simulink model "H175_PANKL_V1a_controlled_R2022b"  (R2022b)
settings: Solver=ode15s  StartTime=0.0  StopTime=22136  RelTol=1e-3  AbsTol=1e-3
PreLoadFcn:
  | omega_TLU = [1000, 1500, 2000, 2500, 3000, 3500];
  | beta_TLU = linspace(0,1,7);
  | 
  | mdot_TLU = [0.1377    0.1304    0.1187    0.1029    0.0854    0.0658    0.0437
  |     0.2310    0.2183    0.1978    0.1688    0.1400    0.1118    0.0750
  |     0.3298    0.3208    0.2987    0.2677    0.2256    0.1774    0.1194
  |     0.4520    0.4260    0.3825    0.3308    0.2745    0.2227    0.1655
  |     0.5542    0.5353    0.4781    0.4230    0.3477    0.2897    0.2211
  |     0.6197    0.5805    0.5198    0.4516    0.3971    0.3555    0.2825];
  | 
  | eta_TLU = [0.7905    0.8025    0.7998    0.7972    0.7932    0.7882    0.7827
  |     0.7993    0.8239    0.8350    0.8379    0.8197    0.8000    0.7809
  |     0.8011    0.8374    0.8632    0.8827    0.8749    0.8394    0.7948
  |     0.8072    0.8520    0.8814    0.9000    0.8676    0.8356    0.7971
  |     0.8076    0.8271    0.8608    0.8766    0.8529    0.8329    0.7992
  |     0.7949    0.8131    0.8296    0.8243    0.8170    0.8085    0.7972];
  | 
  | pr_TLU = [1.0912    1.1795    1.2293    1.2662    1.2928    1.3108    1.3151
  |     1.1484    1.3081    1.3958    1.4707    1.5136    1.5380    1.5456
  |     1.2830    1.4539    1.5943    1.7042    1.7973    1.8582    1.8799
  |     1.5180    1.8034    1.9693    2.0899    2.1662    2.2027    2.2182
  |     1.8359    2.0956    2.3359    2.4668    2.5687    2.6106    2.6224
  |     2.3061    2.6623    2.8585    2.9837    3.0443    3.0714    3.0869];
values from neighbouring files (symbols this model uses):
  P64_omega_TLU = [44762 68636 92509 110414 125335 137271 146224]    [All_Properties.mat]    (also in PANKL_CMP.mat = [44762 68636 92509 110414 125335 137271 146224 155176.0695 1)
libraries: fl_lib x101, nesl_utility x76, SimscapeFluids_lib x5, slpidlib x3
(part 4 of 4)

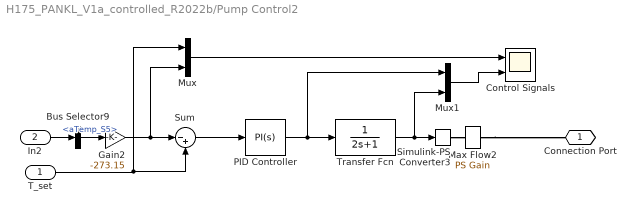
== system H175_PANKL_V1a_controlled_R2022b/Pump Control2 ==
  T_set : Inport
  In2 : Inport  Port=2
  Bus Selector9 : BusSelector  OutputSignals=aTemp_S5
  Control Signals : Scope  NumInputPorts=2
  Gain2 : Gain  Gain=-273.15
  Max Flow2 : fl_lib/Physical Signals/Functions/PS Gain  gain=2 kg/s
  Mux : Mux  Inputs=2
  Mux1 : Mux  Inputs=2
  PID Controller : slpidlib/PID Controller  Controller=PI  Form=Ideal  TimeDomain=Continuous-time  UseExternalTs=off  SampleTime=-1  IntegratorMethod=Forward Euler  FilterMethod=Forward Euler  ControllerParametersSource=internal  P=0.1  I=0.01  UseKiTs=off  D=0  N=100  UseFilter=on  TunerSelectOption=Transfer Function Based (PID Tuner App)  ZeroCross=off  InitialConditionSource=internal  InitialConditionForIntegrator=0  InitialConditionForFilter=0  DifferentiatorICPrevScaledInput=0  ExternalReset=none  TrackingMode=off  Kt=1  LimitOutput=on  SatLimitsSource=internal  UpperSaturationLimit=1  LowerSaturationLimit=0  LinearizeAsGain=on  AntiWindupMode=clamping  Kb=1  LimitIntegrator=off  UpperIntegratorSaturationLimit=inf  LowerIntegratorSaturationLimit=-inf  POutMin=[]  POutMax=[]  IOutMin=[]  IOutMax=[]  DOutMin=[]  DOutMax=[]  NOutMin=[]  NOutMax=[]  SumOutMin=[]  SumOutMax=[]  SaturationOutMin=[]  SaturationOutMax=[]  PParamMin=[]  PParamMax=[]  IParamMin=[]  IParamMax=[]  DParamMin=[]  DParamMax=[]  NParamMin=[]  NParamMax=[]  KbParamMin=[]  KbParamMax=[]  KtParamMin=[]  KtParamMax=[]  KbOutMin=[]  KbOutMax=[]  KtOutMin=[]  KtOutMax=[]  IntegratorOutMin=[]  IntegratorOutMax=[]  FilterOutMin=[]  FilterOutMax=[]  SumI1OutMin=[]  SumI1OutMax=[]  SumI2OutMin=[]  SumI2OutMax=[]  SumI3OutMin=[]  SumI3OutMax=[]  SumI4OutMin=[]  SumI4OutMax=[]  SumDOutMin=[]  SumDOutMax=[]  DifferentiatorOutMin=[]  DifferentiatorOutMax=[]  FilterDiffOutCoefMin=[]  FilterDiffOutCoefMax=[]  ReciprocalOutMin=[]  ReciprocalOutMax=[]  SumDenOutMin=[]  SumDenOutMax=[]  SumNumOutMin=[]  SumNumOutMax=[]  DivideOutMin=[]  DivideOutMax=[]  UdiffTsProdOutMin=[]  UdiffTsProdOutMax=[]  NTsProdOutMin=[]  NTsProdOutMax=[]  UintegralTsProdOutMin=[]  UintegralTsProdOutMax=[]  UngainTsProdOutMin=[]  UngainTsProdOutMax=[]  IntegratorContinuousStateAttributes=''  IntegratorStateMustResolveToSignalObject=off  IntegratorRTWStateStorageClass=Auto  FilterContinuousStateAttributes=''  FilterStateMustResolveToSignalObject=off  FilterRTWStateStorageClass=Auto  ParallelPVariant=Passthrough  IdealPVariant=InternalParameters  IVariant=InternalParameters  DVariant=Disabled  IntegratorVariant=Continuous  SatVariant=Enabled  AWVariant=ContClampingIdeal  PCopyVariant=InternalParamsIdeal  TRVariant=Disabled  FdbkBlocksVariant=Forward  IdealPFdbkVariant=Disabled  SatFdbkVariant=Disabled  DerivativeFilterVariant=Disabled  NVariant=Disabled  NCopyVariant=Disabled_SignalSpec  FilterICVariant=Disabled  IntegratorICVariant=InternalICs  ExternalResetVariant=Disabled  TRSumVariant=Passthrough  SumFdbkVariant=Disabled  SumVariant=Sum_PI  TsampFilterVariant=InternalTs  TsampNgainVariant=Passthrough  TsampIntegralVariant=Disabled_SignalSpec  ExternalSaturationOutDataTypeStr=Inherit: Same as second input
  Simulink-PS Converter3 : nesl_utility/Simulink-PS Converter  PhysicalDomain=network_engine_domain  SubClassName=ps_input  LeftPortType=input  RightPortType=output  PseudoPeriodic=off  Frequencies=[]  NoiseDistribution=none  NoiseParameters=[]  Unit=1  AffineConversion=off  FilteringAndDerivatives=provide  SimscapeFilterOrder=1  InputFilterTimeConstant=0.001  UdotUserProvided=0
  Sum : Sum  Inputs=|-+
  Transfer Fcn : TransferFcn  Denominator=[2 1]
  Connection Port : PMIOPort  Side=Right
  wires:
  Transfer Fcn/1 -> Simulink-PS Converter3/1, Mux1/2
  T_set/1 -> Mux/1, Sum/2
  Gain2/1 -> Sum/1, Mux/2
  Sum/1 -> PID Controller/1
  PID Controller/1 -> Mux1/1, Transfer Fcn/1
  Mux/1 -> Control Signals/1
  Mux1/1 -> Control Signals/2
  Bus Selector9/1 -> Gain2/1  "<aTemp_S5>"
  In2/1 -> Bus Selector9/1
  connections:
  Max Flow2/RConn1 -- Connection Port/RConn1
  Simulink-PS Converter3/RConn1 -- Max Flow2/LConn1

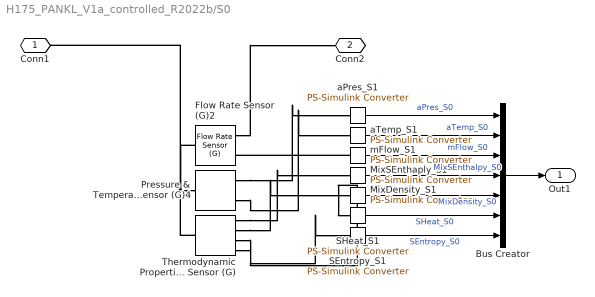
== system H175_PANKL_V1a_controlled_R2022b/S0 ==
  Bus Creator : BusCreator  Inputs=7
  Flow Rate Sensor (G)2 : fl_lib/Gas/Sensors/Flow Rate Sensor (G)  mass_flow_measure=true  volumetric_flow_measure=false  volumetric_flow_conditions=foundation.enum.volumetric_flow_conditions.actual  p_std=0.101325 MPa  T_std=20 degC  energy_flow_measure=false
      settings: InternalSimscapePortConfiguration="{\"Bottom\":[],\"Left\":[{\"id\":\"A\",\"label\":\"A\",\"type\":\"foundation.gas.gas\"}],\"Right\":[{\"id\":\"B\",\"label\":\"B\",\"type\":\"foundation.gas.gas\"},{\"id\":\"M\",\"label\":\"M\",\"type\":\"output\"}],\"Top\":[]}"
  MixDensity_S1 : nesl_utility/PS-Simulink Converter  PhysicalDomain=network_engine_domain  SubClassName=ps_output  LeftPortType=input  RightPortType=output  PseudoPeriodic=off  Frequencies=[]  VectorFormat=inherit  Unit=inherit  AffineConversion=off
  MixSEnthaply_S1 : nesl_utility/PS-Simulink Converter  PhysicalDomain=network_engine_domain  SubClassName=ps_output  LeftPortType=input  RightPortType=output  PseudoPeriodic=off  Frequencies=[]  VectorFormat=inherit  Unit=inherit  AffineConversion=off
  Pressure & Temperature Sensor (G)4 : fl_lib/Gas/Sensors/Pressure & Temperature Sensor (G)  reference=foundation.enum.MeasurementReference.absolute  pressure=true  pressure_spec=foundation.enum.PressureMeasementSpec.Absolute  temperature=true
      settings: InternalSimscapePortConfiguration="{\"Bottom\":[{\"id\":\"T\",\"label\":\"T\",\"type\":\"output\"}],\"Left\":[{\"id\":\"A\",\"label\":\"A\",\"type\":\"foundation.gas.gas\"}],\"Right\":[{\"id\":\"Pa\",\"label\":\"Pa\",\"type\":\"output\"}],\"Top\":[]}"
  SEntropy_S1 : nesl_utility/PS-Simulink Converter  PhysicalDomain=network_engine_domain  SubClassName=ps_output  LeftPortType=input  RightPortType=output  PseudoPeriodic=off  Frequencies=[]  VectorFormat=inherit  Unit=inherit  AffineConversion=off
  SHeat_S1 : nesl_utility/PS-Simulink Converter  PhysicalDomain=network_engine_domain  SubClassName=ps_output  LeftPortType=input  RightPortType=output  PseudoPeriodic=off  Frequencies=[]  VectorFormat=inherit  Unit=inherit  AffineConversion=off
  Thermodynamic Properties Sensor (G) : fl_lib/Gas/Sensors/Thermodynamic Properties Sensor (G)  enthalpy=true  density=true  specific_heat=true  entropy=true  s_std=3.8635 kJ/(K*kg)  p_std=0.101325 MPa  T_std=293.15 K
      settings: InternalSimscapePortConfiguration="{\"Bottom\":[{\"id\":\"CP\",\"label\":\"cp\",\"type\":\"output\"},{\"id\":\"S\",\"label\":\"s\",\"type\":\"output\"}],\"Left\":[{\"id\":\"A\",\"label\":\"A\",\"type\":\"foundation.gas.gas\"}],\"Right\":[{\"id\":\"H\",\"label\":\"h\",\"type\":\"output\"},{\"id\":\"RHO\",\"label\":\"ρ\",\"type\":\"output\"}],\"Top\":[]}"
  aPres_S1 : nesl_utility/PS-Simulink Converter  PhysicalDomain=network_engine_domain  SubClassName=ps_output  LeftPortType=input  RightPortType=output  PseudoPeriodic=off  Frequencies=[]  VectorFormat=inherit  Unit=inherit  AffineConversion=off
  aTemp_S1 : nesl_utility/PS-Simulink Converter  PhysicalDomain=network_engine_domain  SubClassName=ps_output  LeftPortType=input  RightPortType=output  PseudoPeriodic=off  Frequencies=[]  VectorFormat=inherit  Unit=degC  AffineConversion=off
  mFlow_S1 : nesl_utility/PS-Simulink Converter  PhysicalDomain=network_engine_domain  SubClassName=ps_output  LeftPortType=input  RightPortType=output  PseudoPeriodic=off  Frequencies=[]  VectorFormat=inherit  Unit=inherit  AffineConversion=off
  Conn1 : PMIOPort  Side=Left
  Conn2 : PMIOPort  Port=2  Side=Right
  Out1 : Outport
  wires:
  MixDensity_S1/1 -> Bus Creator/5  "MixDensity_S0"
  MixSEnthaply_S1/1 -> Bus Creator/4  "MixSEnthalpy_S0"
  mFlow_S1/1 -> Bus Creator/3  "mFlow_S0"
  Bus Creator/1 -> Out1/1
  aPres_S1/1 -> Bus Creator/1  "aPres_S0"
  SHeat_S1/1 -> Bus Creator/6  "SHeat_S0"
  SEntropy_S1/1 -> Bus Creator/7  "SEntropy_S0"
  aTemp_S1/1 -> Bus Creator/2  "aTemp_S0"
  connections:
  Flow Rate Sensor (G)2/RConn1 -- Conn2/RConn1
  Pressure & Temperature Sensor (G)4/RConn2 -- aTemp_S1/LConn1
  mFlow_S1/LConn1 -- Flow Rate Sensor (G)2/RConn2
  Thermodynamic Properties Sensor (G)/RConn1 -- MixSEnthaply_S1/LConn1
  Thermodynamic Properties Sensor (G)/RConn4 -- SEntropy_S1/LConn1
  Thermodynamic Properties Sensor (G)/RConn2 -- MixDensity_S1/LConn1
  Pressure & Temperature Sensor (G)4/RConn1 -- aPres_S1/LConn1
  Pressure & Temperature Sensor (G)4/LConn1 -- Thermodynamic Properties Sensor (G)/LConn1 -- Conn1/RConn1 -- Flow Rate Sensor (G)2/LConn1
  Thermodynamic Properties Sensor (G)/RConn3 -- SHeat_S1/LConn1

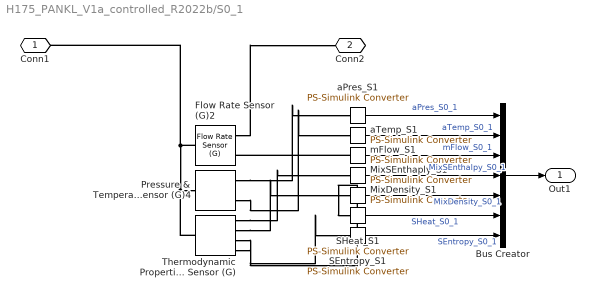
== system H175_PANKL_V1a_controlled_R2022b/S0_1 ==
  Bus Creator : BusCreator  Inputs=7
  Flow Rate Sensor (G)2 : fl_lib/Gas/Sensors/Flow Rate Sensor (G)  mass_flow_measure=true  volumetric_flow_measure=false  volumetric_flow_conditions=foundation.enum.volumetric_flow_conditions.actual  p_std=0.101325 MPa  T_std=20 degC  energy_flow_measure=false
      settings: InternalSimscapePortConfiguration="{\"Bottom\":[],\"Left\":[{\"id\":\"A\",\"label\":\"A\",\"type\":\"foundation.gas.gas\"}],\"Right\":[{\"id\":\"B\",\"label\":\"B\",\"type\":\"foundation.gas.gas\"},{\"id\":\"M\",\"label\":\"M\",\"type\":\"output\"}],\"Top\":[]}"
  MixDensity_S1 : nesl_utility/PS-Simulink Converter  PhysicalDomain=network_engine_domain  SubClassName=ps_output  LeftPortType=input  RightPortType=output  PseudoPeriodic=off  Frequencies=[]  VectorFormat=inherit  Unit=inherit  AffineConversion=off
  MixSEnthaply_S1 : nesl_utility/PS-Simulink Converter  PhysicalDomain=network_engine_domain  SubClassName=ps_output  LeftPortType=input  RightPortType=output  PseudoPeriodic=off  Frequencies=[]  VectorFormat=inherit  Unit=inherit  AffineConversion=off
  Pressure & Temperature Sensor (G)4 : fl_lib/Gas/Sensors/Pressure & Temperature Sensor (G)  reference=foundation.enum.MeasurementReference.absolute  pressure=true  pressure_spec=foundation.enum.PressureMeasementSpec.Absolute  temperature=true
      settings: InternalSimscapePortConfiguration="{\"Bottom\":[{\"id\":\"T\",\"label\":\"T\",\"type\":\"output\"}],\"Left\":[{\"id\":\"A\",\"label\":\"A\",\"type\":\"foundation.gas.gas\"}],\"Right\":[{\"id\":\"Pa\",\"label\":\"Pa\",\"type\":\"output\"}],\"Top\":[]}"
  SEntropy_S1 : nesl_utility/PS-Simulink Converter  PhysicalDomain=network_engine_domain  SubClassName=ps_output  LeftPortType=input  RightPortType=output  PseudoPeriodic=off  Frequencies=[]  VectorFormat=inherit  Unit=inherit  AffineConversion=off
  SHeat_S1 : nesl_utility/PS-Simulink Converter  PhysicalDomain=network_engine_domain  SubClassName=ps_output  LeftPortType=input  RightPortType=output  PseudoPeriodic=off  Frequencies=[]  VectorFormat=inherit  Unit=inherit  AffineConversion=off
  Thermodynamic Properties Sensor (G) : fl_lib/Gas/Sensors/Thermodynamic Properties Sensor (G)  enthalpy=true  density=true  specific_heat=true  entropy=true  s_std=3.8635 kJ/(K*kg)  p_std=0.101325 MPa  T_std=293.15 K
      settings: InternalSimscapePortConfiguration="{\"Bottom\":[{\"id\":\"CP\",\"label\":\"cp\",\"type\":\"output\"},{\"id\":\"S\",\"label\":\"s\",\"type\":\"output\"}],\"Left\":[{\"id\":\"A\",\"label\":\"A\",\"type\":\"foundation.gas.gas\"}],\"Right\":[{\"id\":\"H\",\"label\":\"h\",\"type\":\"output\"},{\"id\":\"RHO\",\"label\":\"ρ\",\"type\":\"output\"}],\"Top\":[]}"
  aPres_S1 : nesl_utility/PS-Simulink Converter  PhysicalDomain=network_engine_domain  SubClassName=ps_output  LeftPortType=input  RightPortType=output  PseudoPeriodic=off  Frequencies=[]  VectorFormat=inherit  Unit=inherit  AffineConversion=off
  aTemp_S1 : nesl_utility/PS-Simulink Converter  PhysicalDomain=network_engine_domain  SubClassName=ps_output  LeftPortType=input  RightPortType=output  PseudoPeriodic=off  Frequencies=[]  VectorFormat=inherit  Unit=degC  AffineConversion=off
  mFlow_S1 : nesl_utility/PS-Simulink Converter  PhysicalDomain=network_engine_domain  SubClassName=ps_output  LeftPortType=input  RightPortType=output  PseudoPeriodic=off  Frequencies=[]  VectorFormat=inherit  Unit=inherit  AffineConversion=off
  Conn1 : PMIOPort  Side=Left
  Conn2 : PMIOPort  Port=2  Side=Right
  Out1 : Outport
  wires:
  MixDensity_S1/1 -> Bus Creator/5  "MixDensity_S0_1"
  MixSEnthaply_S1/1 -> Bus Creator/4  "MixSEnthalpy_S0_1"
  mFlow_S1/1 -> Bus Creator/3  "mFlow_S0_1"
  Bus Creator/1 -> Out1/1
  aPres_S1/1 -> Bus Creator/1  "aPres_S0_1"
  SHeat_S1/1 -> Bus Creator/6  "SHeat_S0_1"
  SEntropy_S1/1 -> Bus Creator/7  "SEntropy_S0_1"
  aTemp_S1/1 -> Bus Creator/2  "aTemp_S0_1"
  connections:
  Flow Rate Sensor (G)2/RConn1 -- Conn2/RConn1
  Pressure & Temperature Sensor (G)4/RConn2 -- aTemp_S1/LConn1
  mFlow_S1/LConn1 -- Flow Rate Sensor (G)2/RConn2
  Thermodynamic Properties Sensor (G)/RConn1 -- MixSEnthaply_S1/LConn1
  Thermodynamic Properties Sensor (G)/RConn4 -- SEntropy_S1/LConn1
  Thermodynamic Properties Sensor (G)/RConn2 -- MixDensity_S1/LConn1
  Pressure & Temperature Sensor (G)4/RConn1 -- aPres_S1/LConn1
  Conn1/RConn1 -- Flow Rate Sensor (G)2/LConn1 -- Pressure & Temperature Sensor (G)4/LConn1 -- Thermodynamic Properties Sensor (G)/LConn1
  Thermodynamic Properties Sensor (G)/RConn3 -- SHeat_S1/LConn1

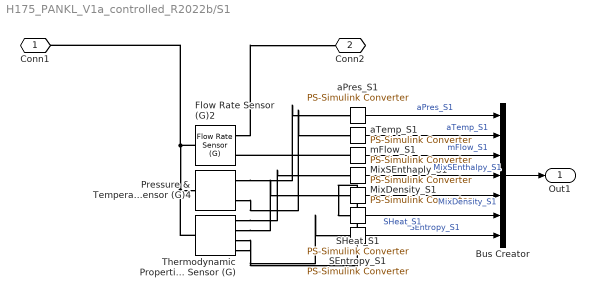
== system H175_PANKL_V1a_controlled_R2022b/S1 ==
  Bus Creator : BusCreator  Inputs=7
  Flow Rate Sensor (G)2 : fl_lib/Gas/Sensors/Flow Rate Sensor (G)  mass_flow_measure=true  volumetric_flow_measure=false  volumetric_flow_conditions=foundation.enum.volumetric_flow_conditions.actual  p_std=0.101325 MPa  T_std=20 degC  energy_flow_measure=false
      settings: InternalSimscapePortConfiguration="{\"Bottom\":[],\"Left\":[{\"id\":\"A\",\"label\":\"A\",\"type\":\"foundation.gas.gas\"}],\"Right\":[{\"id\":\"B\",\"label\":\"B\",\"type\":\"foundation.gas.gas\"},{\"id\":\"M\",\"label\":\"M\",\"type\":\"output\"}],\"Top\":[]}"
  MixDensity_S1 : nesl_utility/PS-Simulink Converter  PhysicalDomain=network_engine_domain  SubClassName=ps_output  LeftPortType=input  RightPortType=output  PseudoPeriodic=off  Frequencies=[]  VectorFormat=inherit  Unit=inherit  AffineConversion=off
  MixSEnthaply_S1 : nesl_utility/PS-Simulink Converter  PhysicalDomain=network_engine_domain  SubClassName=ps_output  LeftPortType=input  RightPortType=output  PseudoPeriodic=off  Frequencies=[]  VectorFormat=inherit  Unit=inherit  AffineConversion=off
  Pressure & Temperature Sensor (G)4 : fl_lib/Gas/Sensors/Pressure & Temperature Sensor (G)  reference=foundation.enum.MeasurementReference.absolute  pressure=true  pressure_spec=foundation.enum.PressureMeasementSpec.Absolute  temperature=true
      settings: InternalSimscapePortConfiguration="{\"Bottom\":[{\"id\":\"T\",\"label\":\"T\",\"type\":\"output\"}],\"Left\":[{\"id\":\"A\",\"label\":\"A\",\"type\":\"foundation.gas.gas\"}],\"Right\":[{\"id\":\"Pa\",\"label\":\"Pa\",\"type\":\"output\"}],\"Top\":[]}"
  SEntropy_S1 : nesl_utility/PS-Simulink Converter  PhysicalDomain=network_engine_domain  SubClassName=ps_output  LeftPortType=input  RightPortType=output  PseudoPeriodic=off  Frequencies=[]  VectorFormat=inherit  Unit=inherit  AffineConversion=off
  SHeat_S1 : nesl_utility/PS-Simulink Converter  PhysicalDomain=network_engine_domain  SubClassName=ps_output  LeftPortType=input  RightPortType=output  PseudoPeriodic=off  Frequencies=[]  VectorFormat=inherit  Unit=inherit  AffineConversion=off
  Thermodynamic Properties Sensor (G) : fl_lib/Gas/Sensors/Thermodynamic Properties Sensor (G)  enthalpy=true  density=true  specific_heat=true  entropy=true  s_std=3.8635 kJ/(K*kg)  p_std=0.101325 MPa  T_std=293.15 K
      settings: InternalSimscapePortConfiguration="{\"Bottom\":[{\"id\":\"CP\",\"label\":\"cp\",\"type\":\"output\"},{\"id\":\"S\",\"label\":\"s\",\"type\":\"output\"}],\"Left\":[{\"id\":\"A\",\"label\":\"A\",\"type\":\"foundation.gas.gas\"}],\"Right\":[{\"id\":\"H\",\"label\":\"h\",\"type\":\"output\"},{\"id\":\"RHO\",\"label\":\"ρ\",\"type\":\"output\"}],\"Top\":[]}"
  aPres_S1 : nesl_utility/PS-Simulink Converter  PhysicalDomain=network_engine_domain  SubClassName=ps_output  LeftPortType=input  RightPortType=output  PseudoPeriodic=off  Frequencies=[]  VectorFormat=inherit  Unit=inherit  AffineConversion=off
  aTemp_S1 : nesl_utility/PS-Simulink Converter  PhysicalDomain=network_engine_domain  SubClassName=ps_output  LeftPortType=input  RightPortType=output  PseudoPeriodic=off  Frequencies=[]  VectorFormat=inherit  Unit=degC  AffineConversion=off
  mFlow_S1 : nesl_utility/PS-Simulink Converter  PhysicalDomain=network_engine_domain  SubClassName=ps_output  LeftPortType=input  RightPortType=output  PseudoPeriodic=off  Frequencies=[]  VectorFormat=inherit  Unit=inherit  AffineConversion=off
  Conn1 : PMIOPort  Side=Left
  Conn2 : PMIOPort  Port=2  Side=Right
  Out1 : Outport
  wires:
  aTemp_S1/1 -> Bus Creator/2  "aTemp_S1"
  SEntropy_S1/1 -> Bus Creator/7  "SEntropy_S1"
  SHeat_S1/1 -> Bus Creator/6  "SHeat_S1"
  aPres_S1/1 -> Bus Creator/1  "aPres_S1"
  Bus Creator/1 -> Out1/1
  mFlow_S1/1 -> Bus Creator/3  "mFlow_S1"
  MixSEnthaply_S1/1 -> Bus Creator/4  "MixSEnthalpy_S1"
  MixDensity_S1/1 -> Bus Creator/5  "MixDensity_S1"
  connections:
  Thermodynamic Properties Sensor (G)/RConn3 -- SHeat_S1/LConn1
  Flow Rate Sensor (G)2/LConn1 -- Conn1/RConn1 -- Thermodynamic Properties Sensor (G)/LConn1 -- Pressure & Temperature Sensor (G)4/LConn1
  Pressure & Temperature Sensor (G)4/RConn1 -- aPres_S1/LConn1
  Thermodynamic Properties Sensor (G)/RConn2 -- MixDensity_S1/LConn1
  Thermodynamic Properties Sensor (G)/RConn4 -- SEntropy_S1/LConn1
  Thermodynamic Properties Sensor (G)/RConn1 -- MixSEnthaply_S1/LConn1
  mFlow_S1/LConn1 -- Flow Rate Sensor (G)2/RConn2
  Pressure & Temperature Sensor (G)4/RConn2 -- aTemp_S1/LConn1
  Flow Rate Sensor (G)2/RConn1 -- Conn2/RConn1

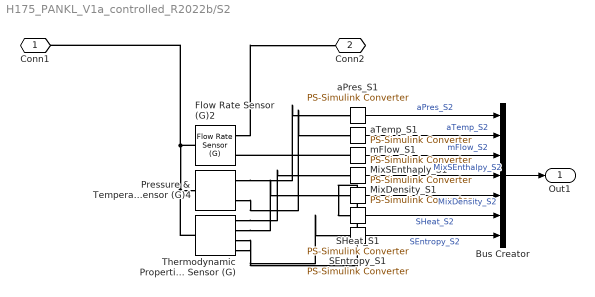
== system H175_PANKL_V1a_controlled_R2022b/S2 ==
  Bus Creator : BusCreator  Inputs=7
  Flow Rate Sensor (G)2 : fl_lib/Gas/Sensors/Flow Rate Sensor (G)  mass_flow_measure=true  volumetric_flow_measure=false  volumetric_flow_conditions=foundation.enum.volumetric_flow_conditions.actual  p_std=0.101325 MPa  T_std=20 degC  energy_flow_measure=false
      settings: InternalSimscapePortConfiguration="{\"Bottom\":[],\"Left\":[{\"id\":\"A\",\"label\":\"A\",\"type\":\"foundation.gas.gas\"}],\"Right\":[{\"id\":\"B\",\"label\":\"B\",\"type\":\"foundation.gas.gas\"},{\"id\":\"M\",\"label\":\"M\",\"type\":\"output\"}],\"Top\":[]}"
  MixDensity_S1 : nesl_utility/PS-Simulink Converter  PhysicalDomain=network_engine_domain  SubClassName=ps_output  LeftPortType=input  RightPortType=output  PseudoPeriodic=off  Frequencies=[]  VectorFormat=inherit  Unit=inherit  AffineConversion=off
  MixSEnthaply_S1 : nesl_utility/PS-Simulink Converter  PhysicalDomain=network_engine_domain  SubClassName=ps_output  LeftPortType=input  RightPortType=output  PseudoPeriodic=off  Frequencies=[]  VectorFormat=inherit  Unit=inherit  AffineConversion=off
  Pressure & Temperature Sensor (G)4 : fl_lib/Gas/Sensors/Pressure & Temperature Sensor (G)  reference=foundation.enum.MeasurementReference.absolute  pressure=true  pressure_spec=foundation.enum.PressureMeasementSpec.Absolute  temperature=true
      settings: InternalSimscapePortConfiguration="{\"Bottom\":[{\"id\":\"T\",\"label\":\"T\",\"type\":\"output\"}],\"Left\":[{\"id\":\"A\",\"label\":\"A\",\"type\":\"foundation.gas.gas\"}],\"Right\":[{\"id\":\"Pa\",\"label\":\"Pa\",\"type\":\"output\"}],\"Top\":[]}"
  SEntropy_S1 : nesl_utility/PS-Simulink Converter  PhysicalDomain=network_engine_domain  SubClassName=ps_output  LeftPortType=input  RightPortType=output  PseudoPeriodic=off  Frequencies=[]  VectorFormat=inherit  Unit=inherit  AffineConversion=off
  SHeat_S1 : nesl_utility/PS-Simulink Converter  PhysicalDomain=network_engine_domain  SubClassName=ps_output  LeftPortType=input  RightPortType=output  PseudoPeriodic=off  Frequencies=[]  VectorFormat=inherit  Unit=inherit  AffineConversion=off
  Thermodynamic Properties Sensor (G) : fl_lib/Gas/Sensors/Thermodynamic Properties Sensor (G)  enthalpy=true  density=true  specific_heat=true  entropy=true  s_std=3.8635 kJ/(K*kg)  p_std=0.101325 MPa  T_std=293.15 K
      settings: InternalSimscapePortConfiguration="{\"Bottom\":[{\"id\":\"CP\",\"label\":\"cp\",\"type\":\"output\"},{\"id\":\"S\",\"label\":\"s\",\"type\":\"output\"}],\"Left\":[{\"id\":\"A\",\"label\":\"A\",\"type\":\"foundation.gas.gas\"}],\"Right\":[{\"id\":\"H\",\"label\":\"h\",\"type\":\"output\"},{\"id\":\"RHO\",\"label\":\"ρ\",\"type\":\"output\"}],\"Top\":[]}"
  aPres_S1 : nesl_utility/PS-Simulink Converter  PhysicalDomain=network_engine_domain  SubClassName=ps_output  LeftPortType=input  RightPortType=output  PseudoPeriodic=off  Frequencies=[]  VectorFormat=inherit  Unit=inherit  AffineConversion=off
  aTemp_S1 : nesl_utility/PS-Simulink Converter  PhysicalDomain=network_engine_domain  SubClassName=ps_output  LeftPortType=input  RightPortType=output  PseudoPeriodic=off  Frequencies=[]  VectorFormat=inherit  Unit=degC  AffineConversion=off
  mFlow_S1 : nesl_utility/PS-Simulink Converter  PhysicalDomain=network_engine_domain  SubClassName=ps_output  LeftPortType=input  RightPortType=output  PseudoPeriodic=off  Frequencies=[]  VectorFormat=inherit  Unit=inherit  AffineConversion=off
  Conn1 : PMIOPort  Side=Left
  Conn2 : PMIOPort  Port=2  Side=Right
  Out1 : Outport
  wires:
  MixDensity_S1/1 -> Bus Creator/5  "MixDensity_S2"
  MixSEnthaply_S1/1 -> Bus Creator/4  "MixSEnthalpy_S2"
  mFlow_S1/1 -> Bus Creator/3  "mFlow_S2"
  Bus Creator/1 -> Out1/1
  aPres_S1/1 -> Bus Creator/1  "aPres_S2"
  SHeat_S1/1 -> Bus Creator/6  "SHeat_S2"
  SEntropy_S1/1 -> Bus Creator/7  "SEntropy_S2"
  aTemp_S1/1 -> Bus Creator/2  "aTemp_S2"
  connections:
  Flow Rate Sensor (G)2/RConn1 -- Conn2/RConn1
  Pressure & Temperature Sensor (G)4/RConn2 -- aTemp_S1/LConn1
  mFlow_S1/LConn1 -- Flow Rate Sensor (G)2/RConn2
  Thermodynamic Properties Sensor (G)/RConn1 -- MixSEnthaply_S1/LConn1
  Thermodynamic Properties Sensor (G)/RConn4 -- SEntropy_S1/LConn1
  Thermodynamic Properties Sensor (G)/RConn2 -- MixDensity_S1/LConn1
  Pressure & Temperature Sensor (G)4/RConn1 -- aPres_S1/LConn1
  Conn1/RConn1 -- Flow Rate Sensor (G)2/LConn1 -- Pressure & Temperature Sensor (G)4/LConn1 -- Thermodynamic Properties Sensor (G)/LConn1
  Thermodynamic Properties Sensor (G)/RConn3 -- SHeat_S1/LConn1

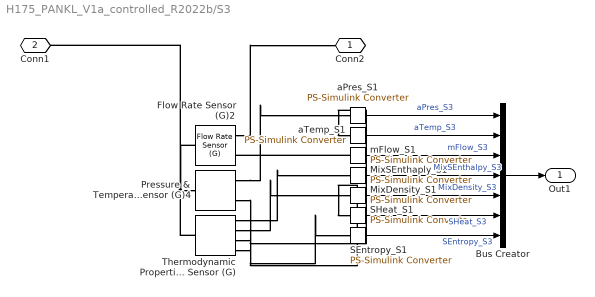
== system H175_PANKL_V1a_controlled_R2022b/S3 ==
  Bus Creator : BusCreator  Inputs=7
  Flow Rate Sensor (G)2 : fl_lib/Gas/Sensors/Flow Rate Sensor (G)  mass_flow_measure=true  volumetric_flow_measure=false  volumetric_flow_conditions=foundation.enum.volumetric_flow_conditions.actual  p_std=0.101325 MPa  T_std=20 degC  energy_flow_measure=false
      settings: InternalSimscapePortConfiguration="{\"Bottom\":[],\"Left\":[{\"id\":\"A\",\"label\":\"A\",\"type\":\"foundation.gas.gas\"}],\"Right\":[{\"id\":\"B\",\"label\":\"B\",\"type\":\"foundation.gas.gas\"},{\"id\":\"M\",\"label\":\"M\",\"type\":\"output\"}],\"Top\":[]}"
  MixDensity_S1 : nesl_utility/PS-Simulink Converter  PhysicalDomain=network_engine_domain  SubClassName=ps_output  LeftPortType=input  RightPortType=output  PseudoPeriodic=off  Frequencies=[]  VectorFormat=inherit  Unit=inherit  AffineConversion=off
  MixSEnthaply_S1 : nesl_utility/PS-Simulink Converter  PhysicalDomain=network_engine_domain  SubClassName=ps_output  LeftPortType=input  RightPortType=output  PseudoPeriodic=off  Frequencies=[]  VectorFormat=inherit  Unit=inherit  AffineConversion=off
  Pressure & Temperature Sensor (G)4 : fl_lib/Gas/Sensors/Pressure & Temperature Sensor (G)  reference=foundation.enum.MeasurementReference.absolute  pressure=true  pressure_spec=foundation.enum.PressureMeasementSpec.Absolute  temperature=true
      settings: InternalSimscapePortConfiguration="{\"Bottom\":[{\"id\":\"T\",\"label\":\"T\",\"type\":\"output\"}],\"Left\":[{\"id\":\"A\",\"label\":\"A\",\"type\":\"foundation.gas.gas\"}],\"Right\":[{\"id\":\"Pa\",\"label\":\"Pa\",\"type\":\"output\"}],\"Top\":[]}"
  SEntropy_S1 : nesl_utility/PS-Simulink Converter  PhysicalDomain=network_engine_domain  SubClassName=ps_output  LeftPortType=input  RightPortType=output  PseudoPeriodic=off  Frequencies=[]  VectorFormat=inherit  Unit=inherit  AffineConversion=off
  SHeat_S1 : nesl_utility/PS-Simulink Converter  PhysicalDomain=network_engine_domain  SubClassName=ps_output  LeftPortType=input  RightPortType=output  PseudoPeriodic=off  Frequencies=[]  VectorFormat=inherit  Unit=inherit  AffineConversion=off
  Thermodynamic Properties Sensor (G) : fl_lib/Gas/Sensors/Thermodynamic Properties Sensor (G)  enthalpy=true  density=true  specific_heat=true  entropy=true  s_std=3.8635 kJ/(K*kg)  p_std=0.101325 MPa  T_std=293.15 K
      settings: InternalSimscapePortConfiguration="{\"Bottom\":[{\"id\":\"CP\",\"label\":\"cp\",\"type\":\"output\"},{\"id\":\"S\",\"label\":\"s\",\"type\":\"output\"}],\"Left\":[{\"id\":\"A\",\"label\":\"A\",\"type\":\"foundation.gas.gas\"}],\"Right\":[{\"id\":\"H\",\"label\":\"h\",\"type\":\"output\"},{\"id\":\"RHO\",\"label\":\"ρ\",\"type\":\"output\"}],\"Top\":[]}"
  aPres_S1 : nesl_utility/PS-Simulink Converter  PhysicalDomain=network_engine_domain  SubClassName=ps_output  LeftPortType=input  RightPortType=output  PseudoPeriodic=off  Frequencies=[]  VectorFormat=inherit  Unit=inherit  AffineConversion=off
  aTemp_S1 : nesl_utility/PS-Simulink Converter  PhysicalDomain=network_engine_domain  SubClassName=ps_output  LeftPortType=input  RightPortType=output  PseudoPeriodic=off  Frequencies=[]  VectorFormat=inherit  Unit=degC  AffineConversion=off
  mFlow_S1 : nesl_utility/PS-Simulink Converter  PhysicalDomain=network_engine_domain  SubClassName=ps_output  LeftPortType=input  RightPortType=output  PseudoPeriodic=off  Frequencies=[]  VectorFormat=inherit  Unit=inherit  AffineConversion=off
  Conn2 : PMIOPort  Side=Left
  Conn1 : PMIOPort  Port=2  Side=Right
  Out1 : Outport
  wires:
  aTemp_S1/1 -> Bus Creator/2  "aTemp_S3"
  SEntropy_S1/1 -> Bus Creator/7  "SEntropy_S3"
  SHeat_S1/1 -> Bus Creator/6  "SHeat_S3"
  aPres_S1/1 -> Bus Creator/1  "aPres_S3"
  Bus Creator/1 -> Out1/1
  mFlow_S1/1 -> Bus Creator/3  "mFlow_S3"
  MixSEnthaply_S1/1 -> Bus Creator/4  "MixSEnthalpy_S3"
  MixDensity_S1/1 -> Bus Creator/5  "MixDensity_S3"
  connections:
  Thermodynamic Properties Sensor (G)/RConn3 -- SHeat_S1/LConn1
  Thermodynamic Properties Sensor (G)/LConn1 -- Pressure & Temperature Sensor (G)4/LConn1 -- Flow Rate Sensor (G)2/LConn1 -- Conn1/RConn1
  Pressure & Temperature Sensor (G)4/RConn1 -- aPres_S1/LConn1
  Thermodynamic Properties Sensor (G)/RConn2 -- MixDensity_S1/LConn1
  Thermodynamic Properties Sensor (G)/RConn4 -- SEntropy_S1/LConn1
  Thermodynamic Properties Sensor (G)/RConn1 -- MixSEnthaply_S1/LConn1
  mFlow_S1/LConn1 -- Flow Rate Sensor (G)2/RConn2
  Pressure & Temperature Sensor (G)4/RConn2 -- aTemp_S1/LConn1
  Flow Rate Sensor (G)2/RConn1 -- Conn2/RConn1

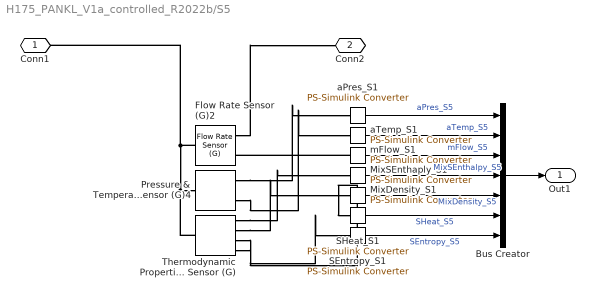
== system H175_PANKL_V1a_controlled_R2022b/S5 ==
  Bus Creator : BusCreator  Inputs=7
  Flow Rate Sensor (G)2 : fl_lib/Gas/Sensors/Flow Rate Sensor (G)  mass_flow_measure=true  volumetric_flow_measure=false  volumetric_flow_conditions=foundation.enum.volumetric_flow_conditions.actual  p_std=0.101325 MPa  T_std=20 degC  energy_flow_measure=false
      settings: InternalSimscapePortConfiguration="{\"Bottom\":[],\"Left\":[{\"id\":\"A\",\"label\":\"A\",\"type\":\"foundation.gas.gas\"}],\"Right\":[{\"id\":\"B\",\"label\":\"B\",\"type\":\"foundation.gas.gas\"},{\"id\":\"M\",\"label\":\"M\",\"type\":\"output\"}],\"Top\":[]}"
  MixDensity_S1 : nesl_utility/PS-Simulink Converter  PhysicalDomain=network_engine_domain  SubClassName=ps_output  LeftPortType=input  RightPortType=output  PseudoPeriodic=off  Frequencies=[]  VectorFormat=inherit  Unit=inherit  AffineConversion=off
  MixSEnthaply_S1 : nesl_utility/PS-Simulink Converter  PhysicalDomain=network_engine_domain  SubClassName=ps_output  LeftPortType=input  RightPortType=output  PseudoPeriodic=off  Frequencies=[]  VectorFormat=inherit  Unit=inherit  AffineConversion=off
  Pressure & Temperature Sensor (G)4 : fl_lib/Gas/Sensors/Pressure & Temperature Sensor (G)  reference=foundation.enum.MeasurementReference.absolute  pressure=true  pressure_spec=foundation.enum.PressureMeasementSpec.Absolute  temperature=true
      settings: InternalSimscapePortConfiguration="{\"Bottom\":[{\"id\":\"T\",\"label\":\"T\",\"type\":\"output\"}],\"Left\":[{\"id\":\"A\",\"label\":\"A\",\"type\":\"foundation.gas.gas\"}],\"Right\":[{\"id\":\"Pa\",\"label\":\"Pa\",\"type\":\"output\"}],\"Top\":[]}"
  SEntropy_S1 : nesl_utility/PS-Simulink Converter  PhysicalDomain=network_engine_domain  SubClassName=ps_output  LeftPortType=input  RightPortType=output  PseudoPeriodic=off  Frequencies=[]  VectorFormat=inherit  Unit=inherit  AffineConversion=off
  SHeat_S1 : nesl_utility/PS-Simulink Converter  PhysicalDomain=network_engine_domain  SubClassName=ps_output  LeftPortType=input  RightPortType=output  PseudoPeriodic=off  Frequencies=[]  VectorFormat=inherit  Unit=inherit  AffineConversion=off
  Thermodynamic Properties Sensor (G) : fl_lib/Gas/Sensors/Thermodynamic Properties Sensor (G)  enthalpy=true  density=true  specific_heat=true  entropy=true  s_std=3.8635 kJ/(K*kg)  p_std=0.101325 MPa  T_std=293.15 K
      settings: InternalSimscapePortConfiguration="{\"Bottom\":[{\"id\":\"CP\",\"label\":\"cp\",\"type\":\"output\"},{\"id\":\"S\",\"label\":\"s\",\"type\":\"output\"}],\"Left\":[{\"id\":\"A\",\"label\":\"A\",\"type\":\"foundation.gas.gas\"}],\"Right\":[{\"id\":\"H\",\"label\":\"h\",\"type\":\"output\"},{\"id\":\"RHO\",\"label\":\"ρ\",\"type\":\"output\"}],\"Top\":[]}"
  aPres_S1 : nesl_utility/PS-Simulink Converter  PhysicalDomain=network_engine_domain  SubClassName=ps_output  LeftPortType=input  RightPortType=output  PseudoPeriodic=off  Frequencies=[]  VectorFormat=inherit  Unit=inherit  AffineConversion=off
  aTemp_S1 : nesl_utility/PS-Simulink Converter  PhysicalDomain=network_engine_domain  SubClassName=ps_output  LeftPortType=input  RightPortType=output  PseudoPeriodic=off  Frequencies=[]  VectorFormat=inherit  Unit=degC  AffineConversion=off
  mFlow_S1 : nesl_utility/PS-Simulink Converter  PhysicalDomain=network_engine_domain  SubClassName=ps_output  LeftPortType=input  RightPortType=output  PseudoPeriodic=off  Frequencies=[]  VectorFormat=inherit  Unit=inherit  AffineConversion=off
  Conn1 : PMIOPort  Side=Left
  Conn2 : PMIOPort  Port=2  Side=Right
  Out1 : Outport
  wires:
  MixDensity_S1/1 -> Bus Creator/5  "MixDensity_S5"
  MixSEnthaply_S1/1 -> Bus Creator/4  "MixSEnthalpy_S5"
  mFlow_S1/1 -> Bus Creator/3  "mFlow_S5"
  Bus Creator/1 -> Out1/1
  aPres_S1/1 -> Bus Creator/1  "aPres_S5"
  SHeat_S1/1 -> Bus Creator/6  "SHeat_S5"
  SEntropy_S1/1 -> Bus Creator/7  "SEntropy_S5"
  aTemp_S1/1 -> Bus Creator/2  "aTemp_S5"
  connections:
  Flow Rate Sensor (G)2/RConn1 -- Conn2/RConn1
  Pressure & Temperature Sensor (G)4/RConn2 -- aTemp_S1/LConn1
  mFlow_S1/LConn1 -- Flow Rate Sensor (G)2/RConn2
  Thermodynamic Properties Sensor (G)/RConn1 -- MixSEnthaply_S1/LConn1
  Thermodynamic Properties Sensor (G)/RConn4 -- SEntropy_S1/LConn1
  Thermodynamic Properties Sensor (G)/RConn2 -- MixDensity_S1/LConn1
  Pressure & Temperature Sensor (G)4/RConn1 -- aPres_S1/LConn1
  Conn1/RConn1 -- Flow Rate Sensor (G)2/LConn1 -- Pressure & Temperature Sensor (G)4/LConn1 -- Thermodynamic Properties Sensor (G)/LConn1
  Thermodynamic Properties Sensor (G)/RConn3 -- SHeat_S1/LConn1

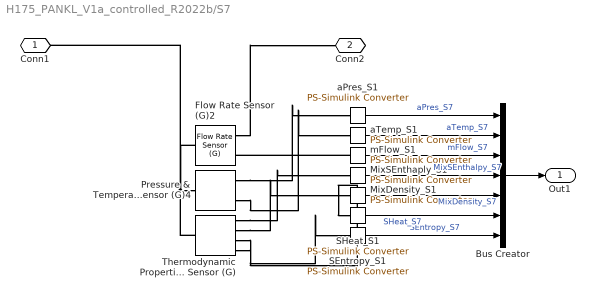
== system H175_PANKL_V1a_controlled_R2022b/S7 ==
  Bus Creator : BusCreator  Inputs=7
  Flow Rate Sensor (G)2 : fl_lib/Gas/Sensors/Flow Rate Sensor (G)  mass_flow_measure=true  volumetric_flow_measure=false  volumetric_flow_conditions=foundation.enum.volumetric_flow_conditions.actual  p_std=0.101325 MPa  T_std=20 degC  energy_flow_measure=false
      settings: InternalSimscapePortConfiguration="{\"Bottom\":[],\"Left\":[{\"id\":\"A\",\"label\":\"A\",\"type\":\"foundation.gas.gas\"}],\"Right\":[{\"id\":\"B\",\"label\":\"B\",\"type\":\"foundation.gas.gas\"},{\"id\":\"M\",\"label\":\"M\",\"type\":\"output\"}],\"Top\":[]}"
  MixDensity_S1 : nesl_utility/PS-Simulink Converter  PhysicalDomain=network_engine_domain  SubClassName=ps_output  LeftPortType=input  RightPortType=output  PseudoPeriodic=off  Frequencies=[]  VectorFormat=inherit  Unit=inherit  AffineConversion=off
  MixSEnthaply_S1 : nesl_utility/PS-Simulink Converter  PhysicalDomain=network_engine_domain  SubClassName=ps_output  LeftPortType=input  RightPortType=output  PseudoPeriodic=off  Frequencies=[]  VectorFormat=inherit  Unit=inherit  AffineConversion=off
  Pressure & Temperature Sensor (G)4 : fl_lib/Gas/Sensors/Pressure & Temperature Sensor (G)  reference=foundation.enum.MeasurementReference.absolute  pressure=true  pressure_spec=foundation.enum.PressureMeasementSpec.Absolute  temperature=true
      settings: InternalSimscapePortConfiguration="{\"Bottom\":[{\"id\":\"T\",\"label\":\"T\",\"type\":\"output\"}],\"Left\":[{\"id\":\"A\",\"label\":\"A\",\"type\":\"foundation.gas.gas\"}],\"Right\":[{\"id\":\"Pa\",\"label\":\"Pa\",\"type\":\"output\"}],\"Top\":[]}"
  SEntropy_S1 : nesl_utility/PS-Simulink Converter  PhysicalDomain=network_engine_domain  SubClassName=ps_output  LeftPortType=input  RightPortType=output  PseudoPeriodic=off  Frequencies=[]  VectorFormat=inherit  Unit=inherit  AffineConversion=off
  SHeat_S1 : nesl_utility/PS-Simulink Converter  PhysicalDomain=network_engine_domain  SubClassName=ps_output  LeftPortType=input  RightPortType=output  PseudoPeriodic=off  Frequencies=[]  VectorFormat=inherit  Unit=inherit  AffineConversion=off
  Thermodynamic Properties Sensor (G) : fl_lib/Gas/Sensors/Thermodynamic Properties Sensor (G)  enthalpy=true  density=true  specific_heat=true  entropy=true  s_std=3.8635 kJ/(K*kg)  p_std=0.101325 MPa  T_std=293.15 K
      settings: InternalSimscapePortConfiguration="{\"Bottom\":[{\"id\":\"CP\",\"label\":\"cp\",\"type\":\"output\"},{\"id\":\"S\",\"label\":\"s\",\"type\":\"output\"}],\"Left\":[{\"id\":\"A\",\"label\":\"A\",\"type\":\"foundation.gas.gas\"}],\"Right\":[{\"id\":\"H\",\"label\":\"h\",\"type\":\"output\"},{\"id\":\"RHO\",\"label\":\"ρ\",\"type\":\"output\"}],\"Top\":[]}"
  aPres_S1 : nesl_utility/PS-Simulink Converter  PhysicalDomain=network_engine_domain  SubClassName=ps_output  LeftPortType=input  RightPortType=output  PseudoPeriodic=off  Frequencies=[]  VectorFormat=inherit  Unit=inherit  AffineConversion=off
  aTemp_S1 : nesl_utility/PS-Simulink Converter  PhysicalDomain=network_engine_domain  SubClassName=ps_output  LeftPortType=input  RightPortType=output  PseudoPeriodic=off  Frequencies=[]  VectorFormat=inherit  Unit=degC  AffineConversion=off
  mFlow_S1 : nesl_utility/PS-Simulink Converter  PhysicalDomain=network_engine_domain  SubClassName=ps_output  LeftPortType=input  RightPortType=output  PseudoPeriodic=off  Frequencies=[]  VectorFormat=inherit  Unit=inherit  AffineConversion=off
  Conn1 : PMIOPort  Side=Left
  Conn2 : PMIOPort  Port=2  Side=Right
  Out1 : Outport
  wires:
  aTemp_S1/1 -> Bus Creator/2  "aTemp_S7"
  SEntropy_S1/1 -> Bus Creator/7  "SEntropy_S7"
  SHeat_S1/1 -> Bus Creator/6  "SHeat_S7"
  aPres_S1/1 -> Bus Creator/1  "aPres_S7"
  Bus Creator/1 -> Out1/1
  mFlow_S1/1 -> Bus Creator/3  "mFlow_S7"
  MixSEnthaply_S1/1 -> Bus Creator/4  "MixSEnthalpy_S7"
  MixDensity_S1/1 -> Bus Creator/5  "MixDensity_S7"
  connections:
  Thermodynamic Properties Sensor (G)/RConn3 -- SHeat_S1/LConn1
  Thermodynamic Properties Sensor (G)/LConn1 -- Pressure & Temperature Sensor (G)4/LConn1 -- Flow Rate Sensor (G)2/LConn1 -- Conn1/RConn1
  Pressure & Temperature Sensor (G)4/RConn1 -- aPres_S1/LConn1
  Thermodynamic Properties Sensor (G)/RConn2 -- MixDensity_S1/LConn1
  Thermodynamic Properties Sensor (G)/RConn4 -- SEntropy_S1/LConn1
  Thermodynamic Properties Sensor (G)/RConn1 -- MixSEnthaply_S1/LConn1
  mFlow_S1/LConn1 -- Flow Rate Sensor (G)2/RConn2
  Pressure & Temperature Sensor (G)4/RConn2 -- aTemp_S1/LConn1
  Flow Rate Sensor (G)2/RConn1 -- Conn2/RConn1

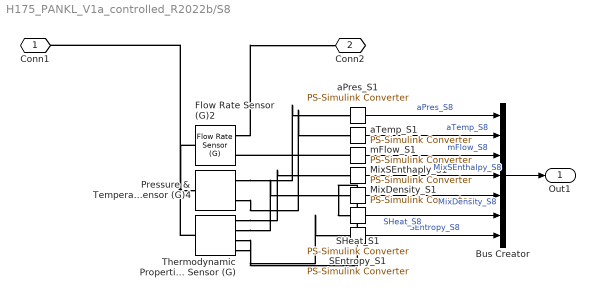
== system H175_PANKL_V1a_controlled_R2022b/S8 ==
  Bus Creator : BusCreator  Inputs=7
  Flow Rate Sensor (G)2 : fl_lib/Gas/Sensors/Flow Rate Sensor (G)  mass_flow_measure=true  volumetric_flow_measure=false  volumetric_flow_conditions=foundation.enum.volumetric_flow_conditions.actual  p_std=0.101325 MPa  T_std=20 degC  energy_flow_measure=false
      settings: InternalSimscapePortConfiguration="{\"Bottom\":[],\"Left\":[{\"id\":\"A\",\"label\":\"A\",\"type\":\"foundation.gas.gas\"}],\"Right\":[{\"id\":\"B\",\"label\":\"B\",\"type\":\"foundation.gas.gas\"},{\"id\":\"M\",\"label\":\"M\",\"type\":\"output\"}],\"Top\":[]}"
  MixDensity_S1 : nesl_utility/PS-Simulink Converter  PhysicalDomain=network_engine_domain  SubClassName=ps_output  LeftPortType=input  RightPortType=output  PseudoPeriodic=off  Frequencies=[]  VectorFormat=inherit  Unit=inherit  AffineConversion=off
  MixSEnthaply_S1 : nesl_utility/PS-Simulink Converter  PhysicalDomain=network_engine_domain  SubClassName=ps_output  LeftPortType=input  RightPortType=output  PseudoPeriodic=off  Frequencies=[]  VectorFormat=inherit  Unit=inherit  AffineConversion=off
  Pressure & Temperature Sensor (G)4 : fl_lib/Gas/Sensors/Pressure & Temperature Sensor (G)  reference=foundation.enum.MeasurementReference.absolute  pressure=true  pressure_spec=foundation.enum.PressureMeasementSpec.Absolute  temperature=true
      settings: InternalSimscapePortConfiguration="{\"Bottom\":[{\"id\":\"T\",\"label\":\"T\",\"type\":\"output\"}],\"Left\":[{\"id\":\"A\",\"label\":\"A\",\"type\":\"foundation.gas.gas\"}],\"Right\":[{\"id\":\"Pa\",\"label\":\"Pa\",\"type\":\"output\"}],\"Top\":[]}"
  SEntropy_S1 : nesl_utility/PS-Simulink Converter  PhysicalDomain=network_engine_domain  SubClassName=ps_output  LeftPortType=input  RightPortType=output  PseudoPeriodic=off  Frequencies=[]  VectorFormat=inherit  Unit=inherit  AffineConversion=off
  SHeat_S1 : nesl_utility/PS-Simulink Converter  PhysicalDomain=network_engine_domain  SubClassName=ps_output  LeftPortType=input  RightPortType=output  PseudoPeriodic=off  Frequencies=[]  VectorFormat=inherit  Unit=inherit  AffineConversion=off
  Thermodynamic Properties Sensor (G) : fl_lib/Gas/Sensors/Thermodynamic Properties Sensor (G)  enthalpy=true  density=true  specific_heat=true  entropy=true  s_std=3.8635 kJ/(K*kg)  p_std=0.101325 MPa  T_std=293.15 K
      settings: InternalSimscapePortConfiguration="{\"Bottom\":[{\"id\":\"CP\",\"label\":\"cp\",\"type\":\"output\"},{\"id\":\"S\",\"label\":\"s\",\"type\":\"output\"}],\"Left\":[{\"id\":\"A\",\"label\":\"A\",\"type\":\"foundation.gas.gas\"}],\"Right\":[{\"id\":\"H\",\"label\":\"h\",\"type\":\"output\"},{\"id\":\"RHO\",\"label\":\"ρ\",\"type\":\"output\"}],\"Top\":[]}"
  aPres_S1 : nesl_utility/PS-Simulink Converter  PhysicalDomain=network_engine_domain  SubClassName=ps_output  LeftPortType=input  RightPortType=output  PseudoPeriodic=off  Frequencies=[]  VectorFormat=inherit  Unit=inherit  AffineConversion=off
  aTemp_S1 : nesl_utility/PS-Simulink Converter  PhysicalDomain=network_engine_domain  SubClassName=ps_output  LeftPortType=input  RightPortType=output  PseudoPeriodic=off  Frequencies=[]  VectorFormat=inherit  Unit=degC  AffineConversion=off
  mFlow_S1 : nesl_utility/PS-Simulink Converter  PhysicalDomain=network_engine_domain  SubClassName=ps_output  LeftPortType=input  RightPortType=output  PseudoPeriodic=off  Frequencies=[]  VectorFormat=inherit  Unit=inherit  AffineConversion=off
  Conn1 : PMIOPort  Side=Left
  Conn2 : PMIOPort  Port=2  Side=Right
  Out1 : Outport
  wires:
  aTemp_S1/1 -> Bus Creator/2  "aTemp_S8"
  SEntropy_S1/1 -> Bus Creator/7  "SEntropy_S8"
  SHeat_S1/1 -> Bus Creator/6  "SHeat_S8"
  aPres_S1/1 -> Bus Creator/1  "aPres_S8"
  Bus Creator/1 -> Out1/1
  mFlow_S1/1 -> Bus Creator/3  "mFlow_S8"
  MixSEnthaply_S1/1 -> Bus Creator/4  "MixSEnthalpy_S8"
  MixDensity_S1/1 -> Bus Creator/5  "MixDensity_S8"
  connections:
  Thermodynamic Properties Sensor (G)/RConn3 -- SHeat_S1/LConn1
  Thermodynamic Properties Sensor (G)/LConn1 -- Pressure & Temperature Sensor (G)4/LConn1 -- Flow Rate Sensor (G)2/LConn1 -- Conn1/RConn1
  Pressure & Temperature Sensor (G)4/RConn1 -- aPres_S1/LConn1
  Thermodynamic Properties Sensor (G)/RConn2 -- MixDensity_S1/LConn1
  Thermodynamic Properties Sensor (G)/RConn4 -- SEntropy_S1/LConn1
  Thermodynamic Properties Sensor (G)/RConn1 -- MixSEnthaply_S1/LConn1
  mFlow_S1/LConn1 -- Flow Rate Sensor (G)2/RConn2
  Pressure & Temperature Sensor (G)4/RConn2 -- aTemp_S1/LConn1
  Flow Rate Sensor (G)2/RConn1 -- Conn2/RConn1

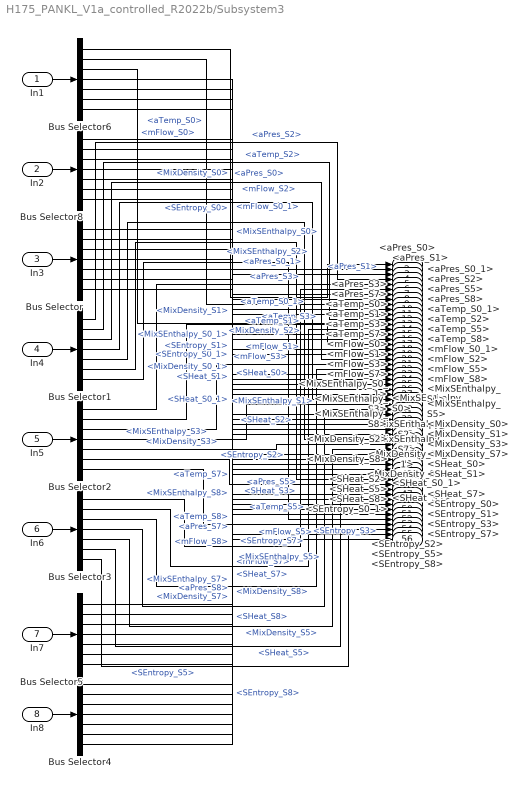
== system H175_PANKL_V1a_controlled_R2022b/Subsystem3 ==
  In1 : Inport
  In2 : Inport  Port=2
  In3 : Inport  Port=3
  In4 : Inport  Port=4
  In5 : Inport  Port=5
  In6 : Inport  Port=6
  In7 : Inport  Port=7
  In8 : Inport  Port=8
  Bus Selector : BusSelector  OutputSignals=aPres_S1,aTemp_S1,mFlow_S1,MixSEnthalpy_S1,MixDensity_S1,SHeat_S1,SEntropy_S1
  Bus Selector1 : BusSelector  OutputSignals=aPres_S2,aTemp_S2,mFlow_S2,MixSEnthalpy_S2,MixDensity_S2,SHeat_S2,SEntropy_S2
  Bus Selector2 : BusSelector  OutputSignals=aPres_S3,aTemp_S3,mFlow_S3,MixSEnthalpy_S3,MixDensity_S3,SHeat_S3,SEntropy_S3
  Bus Selector3 : BusSelector  OutputSignals=aPres_S5,aTemp_S5,mFlow_S5,MixSEnthalpy_S5,MixDensity_S5,SHeat_S5,SEntropy_S5
  Bus Selector4 : BusSelector  OutputSignals=aPres_S8,aTemp_S8,mFlow_S8,MixSEnthalpy_S8,MixDensity_S8,SHeat_S8,SEntropy_S8
  Bus Selector5 : BusSelector  OutputSignals=aPres_S7,aTemp_S7,mFlow_S7,MixSEnthalpy_S7,MixDensity_S7,SHeat_S7,SEntropy_S7
  Bus Selector6 : BusSelector  OutputSignals=aPres_S0,aTemp_S0,mFlow_S0,MixSEnthalpy_S0,MixDensity_S0,SHeat_S0,SEntropy_S0
  Bus Selector8 : BusSelector  OutputSignals=aPres_S0_1,aTemp_S0_1,mFlow_S0_1,MixSEnthalpy_S0_1,MixDensity_S0_1,SHeat_S0_1,SEntropy_S0_1
  <aPres_S0> : Outport
  <aPres_S0_1> : Outport  Port=2
  <aPres_S1> : Outport  Port=3
  <aPres_S2> : Outport  Port=4
  <aPres_S3> : Outport  Port=5
  <aPres_S5> : Outport  Port=6
  <aPres_S7> : Outport  Port=7
  <aPres_S8> : Outport  Port=8
  <aTemp_S0> : Outport  Port=9
  <aTemp_S0_1> : Outport  Port=10
  <aTemp_S1> : Outport  Port=11
  <aTemp_S2> : Outport  Port=12
  <aTemp_S3> : Outport  Port=13
  <aTemp_S5> : Outport  Port=14
  <aTemp_S7> : Outport  Port=15
  <aTemp_S8> : Outport  Port=16
  <mFlow_S0> : Outport  Port=17
  <mFlow_S0_1> : Outport  Port=18
  <mFlow_S1> : Outport  Port=19
  <mFlow_S2> : Outport  Port=20
  <mFlow_S3> : Outport  Port=21
  <mFlow_S5> : Outport  Port=22
  <mFlow_S7> : Outport  Port=23
  <mFlow_S8> : Outport  Port=24
  <MixSEnthalpy_S0> : Outport  Port=25
  <MixSEnthalpy_S0_1> : Outport  Port=26
  <MixSEnthalpy_S1> : Outport  Port=27
  <MixSEnthalpy_S2> : Outport  Port=28
  <MixSEnthalpy_S3> : Outport  Port=29
  <MixSEnthalpy_S5> : Outport  Port=30
  <MixSEnthalpy_S7> : Outport  Port=31
  <MixSEnthalpy_S8> : Outport  Port=32
  <MixDensity_S0> : Outport  Port=33
  <MixDensity_S0_1> : Outport  Port=34
  <MixDensity_S1> : Outport  Port=35
  <MixDensity_S2> : Outport  Port=36
  <MixDensity_S3> : Outport  Port=37
  <MixDensity_S5> : Outport  Port=38
  <MixDensity_S7> : Outport  Port=39
  <MixDensity_S8> : Outport  Port=40
  <SHeat_S0> : Outport  Port=41
  <SHeat_S0_1> : Outport  Port=42
  <SHeat_S1> : Outport  Port=43
  <SHeat_S2> : Outport  Port=44
  <SHeat_S3> : Outport  Port=45
  <SHeat_S5> : Outport  Port=46
  <SHeat_S7> : Outport  Port=47
  <SHeat_S8> : Outport  Port=48
  <SEntropy_S0> : Outport  Port=49
  <SEntropy_S0_1> : Outport  Port=50
  <SEntropy_S1> : Outport  Port=51
  <SEntropy_S2> : Outport  Port=52
  <SEntropy_S3> : Outport  Port=53
  <SEntropy_S5> : Outport  Port=54
  <SEntropy_S7> : Outport  Port=55
  <SEntropy_S8> : Outport  Port=56
  wires:
  Bus Selector/5 -> <MixDensity_S1>/1  "<MixDensity_S1>"
  Bus Selector4/2 -> <aTemp_S8>/1  "<aTemp_S8>"
  Bus Selector2/3 -> <mFlow_S3>/1  "<mFlow_S3>"
  Bus Selector1/4 -> <MixSEnthalpy_S2>/1  "<MixSEnthalpy_S2>"
  Bus Selector4/6 -> <SHeat_S8>/1  "<SHeat_S8>"
  Bus Selector6/2 -> <aTemp_S0>/1  "<aTemp_S0>"
  In2/1 -> Bus Selector8/1
  Bus Selector8/4 -> <MixSEnthalpy_S0_1>/1  "<MixSEnthalpy_S0_1>"
  Bus Selector4/7 -> <SEntropy_S8>/1  "<SEntropy_S8>"
  Bus Selector8/6 -> <SHeat_S0_1>/1  "<SHeat_S0_1>"
  Bus Selector2/4 -> <MixSEnthalpy_S3>/1  "<MixSEnthalpy_S3>"
  Bus Selector/4 -> <MixSEnthalpy_S1>/1  "<MixSEnthalpy_S1>"
  Bus Selector8/7 -> <SEntropy_S0_1>/1  "<SEntropy_S0_1>"
  Bus Selector4/3 -> <mFlow_S8>/1  "<mFlow_S8>"
  Bus Selector4/5 -> <MixDensity_S8>/1  "<MixDensity_S8>"
  Bus Selector2/5 -> <MixDensity_S3>/1  "<MixDensity_S3>"
  Bus Selector8/5 -> <MixDensity_S0_1>/1  "<MixDensity_S0_1>"
  In4/1 -> Bus Selector1/1
  Bus Selector/3 -> <mFlow_S1>/1  "<mFlow_S1>"
  Bus Selector1/7 -> <SEntropy_S2>/1  "<SEntropy_S2>"
  Bus Selector1/2 -> <aTemp_S2>/1  "<aTemp_S2>"
  Bus Selector5/6 -> <SHeat_S7>/1  "<SHeat_S7>"
  In8/1 -> Bus Selector4/1
  Bus Selector4/4 -> <MixSEnthalpy_S8>/1  "<MixSEnthalpy_S8>"
  In3/1 -> Bus Selector/1
  Bus Selector5/5 -> <MixDensity_S7>/1  "<MixDensity_S7>"
  Bus Selector2/2 -> <aTemp_S3>/1  "<aTemp_S3>"
  Bus Selector8/2 -> <aTemp_S0_1>/1  "<aTemp_S0_1>"
  Bus Selector3/2 -> <aTemp_S5>/1  "<aTemp_S5>"
  Bus Selector5/1 -> <aPres_S7>/1  "<aPres_S7>"
  In5/1 -> Bus Selector2/1
  Bus Selector5/4 -> <MixSEnthalpy_S7>/1  "<MixSEnthalpy_S7>"
  Bus Selector5/3 -> <mFlow_S7>/1  "<mFlow_S7>"
  Bus Selector5/2 -> <aTemp_S7>/1  "<aTemp_S7>"
  Bus Selector3/7 -> <SEntropy_S5>/1  "<SEntropy_S5>"
  Bus Selector/7 -> <SEntropy_S1>/1  "<SEntropy_S1>"
  In1/1 -> Bus Selector6/1
  Bus Selector6/1 -> <aPres_S0>/1  "<aPres_S0>"
  Bus Selector1/3 -> <mFlow_S2>/1  "<mFlow_S2>"
  Bus Selector6/5 -> <MixDensity_S0>/1  "<MixDensity_S0>"
  Bus Selector/6 -> <SHeat_S1>/1  "<SHeat_S1>"
  Bus Selector3/3 -> <mFlow_S5>/1  "<mFlow_S5>"
  Bus Selector2/7 -> <SEntropy_S3>/1  "<SEntropy_S3>"
  Bus Selector5/7 -> <SEntropy_S7>/1  "<SEntropy_S7>"
  Bus Selector2/6 -> <SHeat_S3>/1  "<SHeat_S3>"
  Bus Selector3/5 -> <MixDensity_S5>/1  "<MixDensity_S5>"
  Bus Selector2/1 -> <aPres_S3>/1  "<aPres_S3>"
  In7/1 -> Bus Selector5/1
  Bus Selector/2 -> <aTemp_S1>/1  "<aTemp_S1>"
  Bus Selector8/1 -> <aPres_S0_1>/1  "<aPres_S0_1>"
  Bus Selector6/4 -> <MixSEnthalpy_S0>/1  "<MixSEnthalpy_S0>"
  Bus Selector1/1 -> <aPres_S2>/1  "<aPres_S2>"
  Bus Selector8/3 -> <mFlow_S0_1>/1  "<mFlow_S0_1>"
  Bus Selector3/4 -> <MixSEnthalpy_S5>/1  "<MixSEnthalpy_S5>"
  Bus Selector/1 -> <aPres_S1>/1  "<aPres_S1>"
  Bus Selector1/5 -> <MixDensity_S2>/1  "<MixDensity_S2>"
  Bus Selector6/3 -> <mFlow_S0>/1  "<mFlow_S0>"
  Bus Selector3/6 -> <SHeat_S5>/1  "<SHeat_S5>"
  Bus Selector1/6 -> <SHeat_S2>/1  "<SHeat_S2>"
  Bus Selector3/1 -> <aPres_S5>/1  "<aPres_S5>"
  Bus Selector4/1 -> <aPres_S8>/1  "<aPres_S8>"
  Bus Selector6/7 -> <SEntropy_S0>/1  "<SEntropy_S0>"
  In6/1 -> Bus Selector3/1
  Bus Selector6/6 -> <SHeat_S0>/1  "<SHeat_S0>"
